simulink model "sldemo_foucault_vr"  (R2019b)
settings: Solver=ode23t  StartTime=0.0  StopTime=3600  FixedStep=.1  MaxStep=72  RelTol=1e-5  EnableMultiTasking=on
PreLoadFcn:
  | %SLDEMO_FOUCAULT_DATA
  | %
  | % Contains initialization data for the foucault pendulum model
  | %
  | % See also: SLDEMO_FOUCAULT, SLDEMO_FOUCAULT, SLDEMO_FOUCAULT_ANIMATE
  | 
  | g = 9.83;          % acceleration of gravity (m/sec^2)
  | L = 67;            % pendulum length (m)
  | initial_x = 8; % initial x coordinate (m)
  | initial_y = 0;     % initial y coordinate (m)
  | initial_xdot = 0;  % initial x velocity (m/sec)
  | initial_ydot = 0;  % initial y velocity (m/sec)
  | Omega=2*pi/86400;  % Earth's angular velocity of rotation about its axis (rad/sec)
  | % In contrast to original demo slemo_foucault,
  | % lambda is here defined directly in the model
  | % lambda=48.85/180*pi;  % latitude in (rad)
libraries: vrlib x6, simulink_extras x2
Description:
  | Foucault Pendulum Model with VRML Visualization
  | 
  | This model solves the differential equations for the Foucault Pendulum problem
  | and displays the pendulum bob movement in the VRML scene. You can modify
  | the Pendulum location by changing the Latitude / Longitude constant values
  | in the model and other parameters (g, \Omega, L and initial conditions)
  | in MATLAB(R) workspace.
  | 
  | There are two VRML scenes associated with this model. The first scene
  | shows the Foucault pendulum itself, the second shows geographical position
  | of the pendulum on the Earth. During the simulation, two arrow markers
  | indicate the current and the initial position of the pendulum in the Earth
  | coordinate system.
settings Model: ExtModeAutoUpdateStatusClock=off  Creator=The MathWorks, Inc.  LastModifiedBy=The MathWorks, Inc.
settings DataIOCC: SaveFormat=StructureWithTime  SaveOutput=off  SaveTime=off  SignalLoggingName=sldemo_foucault_output
settings OptimizationCC: ExpressionDepthLimit=2147483647  InitFltsAndDblsToZero=on  EfficientMapNaN2IntZero=off  LifeSpan=inf
settings DebuggingCC: SaveWithParameterizedLinksMsg=none  UnderspecifiedInitializationDetection=Classic  MergeDetectMultiDrivingBlocksExec=none  SignalResolutionControl=TryResolveAllWithWarning  SolverPrmCheckMsg=warning  FcnCallInpInsideContextMsg=warning  StateNameClashWarn=warning  SFUnexpectedBacktrackingDiag=warning  SFNoUnconditionalDefaultTransitionDiag=warning  SFExecutionAtInitializationDiag=none  ArithmeticOperatorsInVariantConditions=warning
settings HardwareCC: ProdBitPerPointer=32  ProdBitPerSizeT=32  ProdBitPerPtrDiffT=32  ProdLargestAtomicFloat=None  ProdIntDivRoundTo=Undefined  ProdEndianess=Unspecified  ProdWordSize=32  ProdHWDeviceType=32-bit Generic
settings ModelReferenceCC: PropagateSignalLabelsOutOfModel=off
settings SFSimCC: SimUseLocalCustomCode=off  CustomCodeUndefinedFunction=UseInterfaceOnly
settings RTWCC: RTWUseLocalCustomCode=off
settings CodeAppCC: StateflowObjectComments=on
settings GRTTargetCC: TargetFcnLib=ansi_tfl_tmw.mat  TargetLangStandard=C89/C90 (ANSI)  GeneratePreprocessorConditionals=Disable all  CombineOutputUpdateFcns=off  GRTInterface=on
settings ConfigComp: CovMetricSettings=dw  CovHtmlReporting=on  CovSaveCumulativeToWorkspaceVar=on  CovSaveSingleToWorkspaceVar=on  CovExternalEMLEnable=off

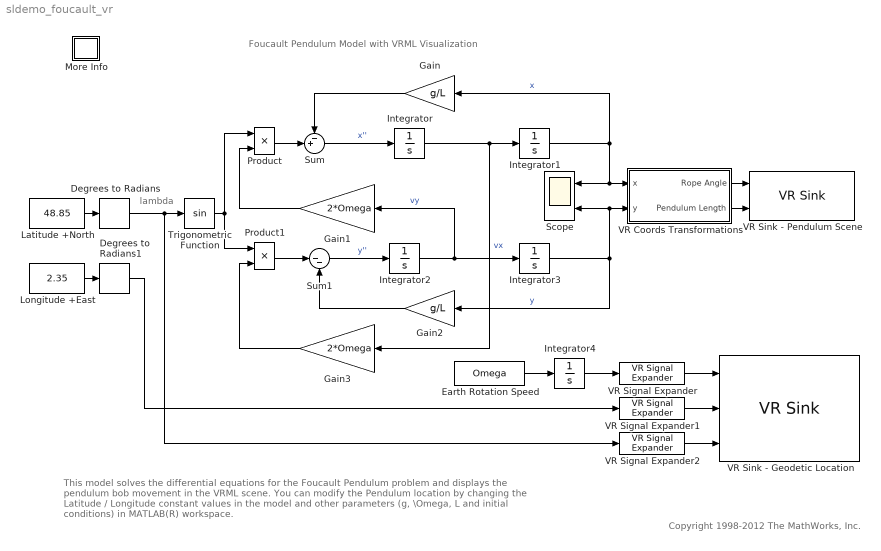
== system sldemo_foucault_vr ==
  note: This model solves the differential equations for the Foucault Pendulum problem
      | and displays the pendulum bob movement in the VRML scene. You can modify the
      | Pendulum location by changing the Latitude / Longitude constant values in the model
      | and other parameters (g, \Omega, L and initial conditions) in MATLAB(R) workspace.
  note: Foucault Pendulum Model with VRML Visualization
  note: lambda
  note: Copyright 1998-2012 The MathWorks, Inc.
  Degrees to Radians : simulink_extras/Transformations/Degrees to Radians
  Degrees to Radians1 : simulink_extras/Transformations/Degrees to Radians
  Earth Rotation Speed : Constant  Value=Omega
  Gain : Gain  Gain=g/L
  Gain1 : Gain  Gain=2*Omega
  Gain2 : Gain  Gain=g/L
  Gain3 : Gain  Gain=2*Omega
  Integrator : Integrator  InitialCondition=initial_xdot
  Integrator1 : Integrator  InitialCondition=initial_x
  Integrator2 : Integrator  InitialCondition=initial_ydot
  Integrator3 : Integrator  InitialCondition=initial_y
  Integrator4 : Integrator
  Latitude +North : Constant  Value=48.85
  Longitude +East : Constant  Value=2.35
  More Info : Subsystem
      settings: OpenFcn=showExample('simulink_general/sldemo_foucault_vrExample')
      mask Display: disp('?')
  Product : Product  RndMeth=Zero
  Product1 : Product  RndMeth=Zero
  Scope : Scope  NumInputPorts=2
  Sum : Sum  Inputs=-+|
  Sum1 : Sum  Inputs=|--
  Trigonometric Function : Trigonometry
  VR Coords Transformations : Subsystem
  VR Signal Expander : vrlib/VR Signal Expander  outwidth=4  outidx=[4]
      settings: SourceProductName=Simulink
  VR Signal Expander1 : vrlib/VR Signal Expander  outwidth=4  outidx=[4]
      settings: SourceProductName=Simulink
  VR Signal Expander2 : vrlib/VR Signal Expander  outwidth=4  outidx=[4]
      settings: SourceProductName=Simulink
  VR Sink - Geodetic Location : vrlib/VR Sink  InstantiateOnLoad=on  SampleTime=0.5  ViewEnable=on  RemoteChange=off  RemoteView=on  FieldsWritten=Earth.rotation.4.1.double#Marker_Rot_Long.rotation.4.1.double#Marker_Rot_Lat.rotation.4.1.double  WorldFileName=foucault_earth.wrl  WorldDescription=The Earth with Foucault Pendulum Location Marker  AutoView=on  VideoDimensions=[]  AllowVariableSize=off  FigureProperties="{'Position', 'Name', 'Viewpoint', 'CameraBound', 'CameraDirection', 'CameraPosition', 'CameraUpVector', 'ZoomFactor', 'Antialiasing', 'Headlight', 'Lighting', 'NavPanel', 'Sound', 'StatusBar', 'Stereo3D', 'Stereo3DCameraOffset', 'Stereo3DHIT', 'ToolBar', 'Textures', 'Transparency', 'Triad', 'Wireframe', 'NavZones', 'NavMode', 'NavSpeed', 'CaptureFileFormat', 'CaptureFileName', 'Record2DCompressMethod', 'Record2DCompressQuality', 'Record2D', 'Record2DFileName', 'Record2DFPS'; [5.2500000000000000e+02   1.4800000000000000e+02   4.1200000000000000e+02   4.9200000000000000e+02], 'The Earth with Foucault Pendulum Location Marker', 'View at 0E 0N', 'on', [0.0000000000000000e+00   0.0000000000000000e+00  -1.0000000000000000e+00], [0.0000000000000000e+00   0.0000000000000000e+00   0.0000000000000000e+00], [0.0000000000000000e+00   1.0000000000000000e+00   0.0000000000000000e+00], [1.0000000000000000e+00], 'off', 'on', 'on', 'none', 'on', 'on', 'off', [1.0000000149011612e-01], [0.0000000000000000e+00], 'on', 'on', 'on', 'none', 'off', 'off', 'examine', 'normal', 'tif', '%f_anim_%n.tif', 'auto', [7.5000000000000000e+01], 'off', '%f_anim_%n.avi', [1.5000000000000000e+01]}"
      settings: SourceProductName=Simulink
  VR Sink - Pendulum Scene : vrlib/VR Sink  InstantiateOnLoad=on  SampleTime=0.1  ViewEnable=on  RemoteChange=off  RemoteView=on  FieldsWritten=Pend.rotation.4.1.double#Pend.translation.3.1.double  WorldFileName=foucault_scene.wrl  WorldDescription=Foucault Pendulum Scene  AutoView=on  VideoDimensions=[]  AllowVariableSize=off  FigureProperties="{'Position', 'Name', 'Viewpoint', 'CameraBound', 'CameraDirection', 'CameraPosition', 'CameraUpVector', 'ZoomFactor', 'Antialiasing', 'Headlight', 'Lighting', 'NavPanel', 'Sound', 'StatusBar', 'Stereo3D', 'Stereo3DCameraOffset', 'Stereo3DHIT', 'ToolBar', 'Textures', 'Transparency', 'Triad', 'Wireframe', 'NavZones', 'NavMode', 'NavSpeed', 'CaptureFileFormat', 'CaptureFileName', 'Record2DCompressMethod', 'Record2DCompressQuality', 'Record2D', 'Record2DFileName', 'Record2DFPS'; [1.1000000000000000e+01   1.4800000000000000e+02   5.0300000000000000e+02   3.4200000000000000e+02], 'Foucault Pendulum Scene', 'View along -X', 'on', [0.0000000000000000e+00   0.0000000000000000e+00  -1.0000000000000000e+00], [0.0000000000000000e+00   0.0000000000000000e+00   0.0000000000000000e+00], [0.0000000000000000e+00   1.0000000000000000e+00   0.0000000000000000e+00], [1.0000000000000000e+00], 'off', 'on', 'on', 'halfbar', 'on', 'off', 'off', [1.0000000149011612e-01], [0.0000000000000000e+00], 'on', 'on', 'on', 'none', 'off', 'off', 'examine', 'normal', 'tif', '%f_anim_%n.tif', 'auto', [7.5000000000000000e+01], 'off', '%f_anim_%n.avi', [1.5000000000000000e+01]}"
      settings: SourceProductName=Simulink
  wires:
  Integrator/1 -> Integrator1/1, Gain3/1  "vx"
  Integrator1/1 -> Scope/1, VR Coords Transformations/1(x), Gain/1  "x"
  Sum/1 -> Integrator/1  "x''"
  Gain/1 -> Sum/1
  Integrator2/1 -> Integrator3/1, Gain1/1  "vy"
  Integrator3/1 -> Scope/2, VR Coords Transformations/2(y), Gain2/1  "y"
  Earth Rotation Speed/1 -> Integrator4/1
  Integrator4/1 -> VR Signal Expander/1
  VR Coords Transformations/1(Rope Angle) -> VR Sink - Pendulum Scene/1
  VR Coords Transformations/2(Pendulum Length) -> VR Sink - Pendulum Scene/2
  Latitude +North/1 -> Degrees to Radians/1
  Longitude +East/1 -> Degrees to Radians1/1
  Gain3/1 -> Product1/2
  Gain1/1 -> Product/2
  Degrees to Radians/1 -> Trigonometric Function/1, VR Signal Expander2/1
  Sum1/1 -> Integrator2/1  "y''"
  Gain2/1 -> Sum1/2
  Product1/1 -> Sum1/1
  Product/1 -> Sum/2
  Trigonometric Function/1 -> Product/1, Product1/1
  VR Signal Expander/1 -> VR Sink - Geodetic Location/1
  Degrees to Radians1/1 -> VR Signal Expander1/1
  VR Signal Expander1/1 -> VR Sink - Geodetic Location/2
  VR Signal Expander2/1 -> VR Sink - Geodetic Location/3

== system sldemo_foucault_vr/More Info ==

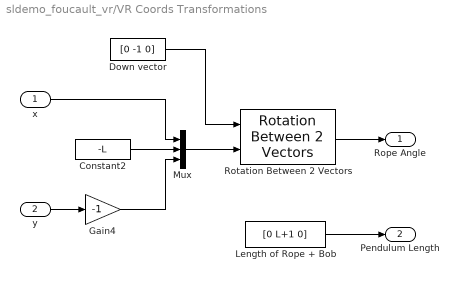
== system sldemo_foucault_vr/VR Coords Transformations ==
  x : Inport
  y : Inport  Port=2
  Constant2 : Constant  Value=-L
  Down vector : Constant  Value=[0 -1 0]
  Gain4 : Gain  Gain=-1
  Length of Rope + Bob : Constant  Value=[0 L+1 0]
  Mux : Mux  Inputs=3
  Rotation Between 2 Vectors : vrlib/Utilities/Rotation Between 2 Vectors
      settings: SourceProductName=Simulink  SourceProductBaseCode=SL
  Rope Angle : Outport  VectorParamsAs1DForOutWhenUnconnected=off
  Pendulum Length : Outport  Port=2  VectorParamsAs1DForOutWhenUnconnected=off
  wires:
  Constant2/1 -> Mux/2
  Down vector/1 -> Rotation Between 2 Vectors/1
  Mux/1 -> Rotation Between 2 Vectors/2
  Gain4/1 -> Mux/3
  x/1 -> Mux/1
  y/1 -> Gain4/1
  Rotation Between 2 Vectors/1 -> Rope Angle/1
  Length of Rope + Bob/1 -> Pendulum Length/1
